simulink model "eq_test"  (Simulink 5.1)
settings: Solver=FixedStepDiscrete  StartTime=0.0  StopTime=inf  RelTol=1e-3
PreLoadFcn:
  | Frame=64;  % number of points in a frame
  | load eq_coefficients;
values from neighbouring files (symbols this model uses):
  D = 2 * W2 * (G01 - sqrt(G00 * G11))    [peq.m]
  num_den_coef = [0.998343259442 -1.98599942437 0.988847189128 1 -1.98599942437 0.98719044857 0.939478810291 -1.81918066061 0.879941563044 1 -1.81918066061 0.819420373336 ... (31 elements, 1x31)]    [eq_coefficients.mat]
undefined symbols (not defined in the file or in its folder): magnitude
libraries: dspsigops x4, dspsigattribs x3, dspsrcs4 x2, dspwin32 x2, dspbuff3 x2, dsparch3 x2, dspxfrm3 x2, dsparch4 x1, simulink x1
settings Model: Creator=aanantha  LastModifiedBy=dbenson  DataSet=allH.mat  SaveTime=off  SaveOutput=off  BooleanDataType=on  ProdHWDeviceType=Microprocessor  RTWOptions="-aEnforceIntegerDowncast=1 -aExtMode=0 -aExtModeTesting=0 -aFoldNonRolledExpr=1 -aForceParamTrailComments=0 -aGenerateComments=1 -aGenerateReport=0 -aIgnoreCustomStorageClasses=1 -aIncDataTypeInIds=0 -aIncHierarchyInIds=0 -aInlineInvariantSignals=0 -aInlinedPrmAccess=\"Literals\" -aLocalBlockOutputs=1 -aLogVarNameModifier=\"rt_\" -aMaxRTWIdLen=31 -aPrefixModelToSubsysFcnNames=1 -aRTWVerbose=1 -aRollThreshold=5 -aShowEliminatedStatements=0"

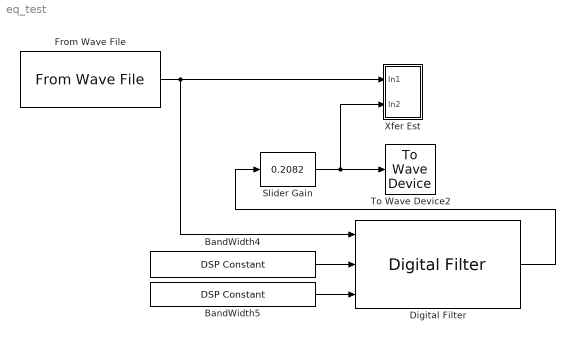
== system eq_test ==
  BandWidth4 : dspsrcs4/DSP Constant  Tag=paramsBlock  Value=conv(conv(num_den_coef(1:3),num_den_coef(7:9)),num_den_coef(13:15))  SampleMode=Discrete  discreteOutput=Sample-based  continuousOutput=Sample-based  sampTime=-1  framePeriod=-1  dataType=Inherit from 'Constant value'  wordLen=16  udDataType=sfix(16)  fracBitsMode=Best precision  numFracBits=15  InterpretAs1D=off  Ts=-1  FramebasedOutput=off
      settings: AttributesFormatString=\n\n\n\n
  BandWidth5 : dspsrcs4/DSP Constant  Tag=paramsBlock  Value=conv(conv(num_den_coef(4:6),num_den_coef(10:12)),num_den_coef(16:18))  SampleMode=Discrete  discreteOutput=Sample-based  continuousOutput=Sample-based  sampTime=-1  framePeriod=-1  dataType=Inherit from 'Constant value'  wordLen=16  udDataType=sfix(16)  fracBitsMode=Best precision  numFracBits=15  InterpretAs1D=off  Ts=-1  FramebasedOutput=off
      settings: AttributesFormatString=\n\n\n\n
  Digital Filter : dsparch4/Digital Filter  TypePopup=IIR (poles & zeros)  IIRFiltStruct=Direct form II transposed  AllPoleFiltStruct=Direct form  FIRFiltStruct=Direct form  CoeffSource=Input port(s)  NumCoeffs=[1 2]  DenCoeffs=[1 0.1]  BiQuadCoeffs=[1 0.3 0.4 1 0.1 0.2]  LatticeCoeffs=[0.2 0.4]  denIgnore=on  FiltPerSampPopup=One filter per frame  IC=0  ICnum=0  ICden=0  roundingMode=Floor  overflowMode=off
  From Wave File : dspwin32/From Wave File  FileName=test_wave.wav  SamplesPerFrame=Frame  MinBufSize=256  dType=Double  bLoop=on  timesToPlay=inf  restartMode=at beginning of next frame (zero pad)  firstSampleOutput=off  lastSampleOutput=off
  Slider Gain : simulink/Math Operations/Slider Gain  low=0.1  gain=0.2082  high=1
  To Wave Device2 : dspwin32/To Wave Device  bufDuration=2  initDelay=0.1  useDefaultDevice=off  userDeviceID=SoundMAX Digital Audio  enable24Bit=off
  Xfer Est : Subsystem  TreatAsAtomicUnit=on  mask(Xfer Scope){ScopeProperties=on, Domain=Frequency, HorizSpan=1, UseBuffer=on, BufferSize=512, Overlap=256, inpFftLenInherit=off, FFTlength=512, numAvg=4, DisplayProperties=off, AxisGrid=on, Memory=off, FrameNumber=on, AxisLegend=off, AxisZoom=off, OpenScopeAtSimStart=on, OpenScopeImmediately=off, FigPos=[484 458 442 191], AxisProperties=off, XUnits=Hertz, XRange=[0...Fs/2], InheritXIncr=on, XIncr=1, XLabel=Samples, YUnits=dB, YMin=-20, YMax=20, YLabel=Magnitude, dB, LineProperties=off, LineDisables=, LineStyles=, LineMarkers=, LineColors=[1 0 0]}
      mask prompts: ScopeProperties "_______ Scope properties _______"; Domain "Input domain:"; HorizSpan "Time display span (number of frames):"; UseBuffer "Buffer input"; BufferSize "Buffer size:"; Overlap "Buffer overlap:"; inpFftLenInherit "Specify FFT length"; FFTlength "FFT length:"; numAvg "Number of spectral averages:"; DisplayProperties "_______ Display properties _______"; AxisGrid "Show grid"; Memory "Persistence"; FrameNumber "Frame number"; AxisLegend "Channel legend"; AxisZoom "Compact display"; OpenScopeAtSimStart "Open scope at start of simulation"; OpenScopeImmediately "Open scope immediately"; FigPos "Scope position:"; AxisProperties "_______ Axis properties _______"; XUnits "Frequency units:"; XRange "Frequency range:"; InheritXIncr "Inherit sample increment from input"; XIncr "Sample time of original time series:"; XLabel "X-axis title:"; YUnits "Amplitude scaling:"; YMin "Minimum Y-limit:"; YMax "Maximum Y-limit:"; YLabel "Y-axis title:"; LineProperties "_______ Line properties _______"; LineDisables "Line visibility:"; LineStyles "Line styles:"; LineMarkers "Line markers:"; LineColors "Line colors:"
      mask help:
      | Computes a non-biased transfer function estimation by using
      | the ratio of the cross spectrum between the excitation and response
      | channels, and the autospectrum of the excitation channel.
      |
      | X= channel 1 = DUT excitation (discrete time random noise is best)
      | Y= channel 2 = DUT response from DUT
      |
      | Displays xfer function magnitude in linear or dB format.
      mask init:
      | [x,y,str] = xferscope1('icon');
      | s = xferscope1('init');
      settings: CopyFcn=sdspfscope2([],[],[],'BlockCopy');  DeleteFcn=sdspfscope2([],[],[],'BlockDelete');  NameChangeFcn=sdspfscope2([],[],[],'NameChange');  RTWSystemCode=Function
      mask Help:
      | Use a broad band discrete time excitation and apply it to both
      | analyzer the upper input port and the (discrete time) Device Under Test input.
      | Connect the discrete time DUT response to the lower input port.
      | Averaging of circa 100 produces good results.
      | 
      | The measurement results will be unbiased as long as the excitation
      | does not have noise which is correlated with noise in the response channel.
      | 
      | 
      | RAB 01/28/02
      mask StyleString: checkbox,popup(Time|Frequency|User-defined),edit,checkbox,edit,edit,checkbox,edit,edit,checkbox,checkbox,checkbox,checkbox,checkbox,checkbox,checkbox,checkbox,edit,checkbox,popup(Hertz|rad/sec),popup([0...Fs/2]|[-Fs/2...Fs/2]|[0...Fs]),checkbox,edit,edit,popup(Magnitude|dB),edit,edit,edit,checkbox,edit,edit,edit,edit
      mask CallbackString: dspblkbfftscope2('dynamic','ScopeProperties')|||dspblkbfftscope2('dynamic','useBuffer');|||dspblkbfftscope2('dynamic','FftLenCheckbox');|||dspblkbfftscope2('dynamic','DisplayProperties');|||||||dspblkbfftscope2('dynamic','OpenScope');||dspblkbfftscope2('dynamic','AxisProperties');|||dspblkbfftscope2('dynamic','InheritXIncr');|||||||dspblkbfftscope2('dynamic','LineProperties');||||
      mask Display: plot(x,y); text(14,20,str);
  wires:
  From Wave File/1 -> Digital Filter/1, Xfer Est/1(In1)
  Slider Gain/1 -> Xfer Est/2(In2), To Wave Device2/1
  BandWidth4/1 -> Digital Filter/2
  BandWidth5/1 -> Digital Filter/3
  Digital Filter/1 -> Slider Gain/1

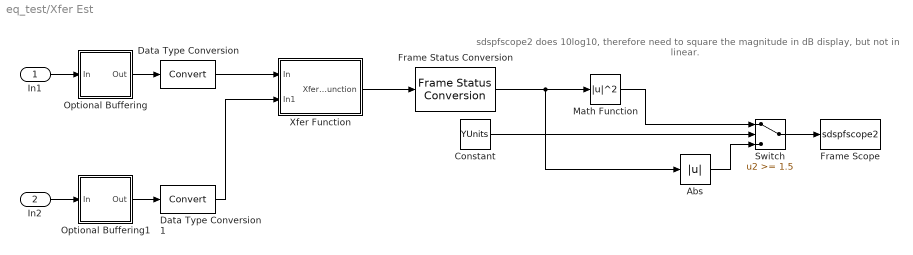
== system eq_test/Xfer Est ==
  note: sdspfscope2 does 10log10, therefore need to square the magnitude in dB
      | display, but not in linear.
  In1 : Inport
  In2 : Inport  Port=2
  Abs : Abs  SaturateOnIntegerOverflow=on
  Constant : Constant  Value=YUnits
  Data Type Conversion : DataTypeConversion  DataType=double  SaturateOnIntegerOverflow=on
  Data Type Conversion1 : DataTypeConversion  DataType=double  SaturateOnIntegerOverflow=on
  Frame Scope : S-Function  FunctionName=sdspfscope2  Parameters=s
  Frame Status Conversion : dspsigattribs/Frame Status Conversion  growRefPort=off  outframe=Sample-based
  Math Function : Math  Operator=magnitude^2
  Optional Buffering : Subsystem  mask(Replaceable Contents){oname=Buffer, osrc=dspbuff3/Buffer, oargs={'N','BufferSize','V','Overlap','ic','0'}, replace=strcmp(UseBuffer,'off')}
      mask prompts: oname "Relative name of blocks to replace:"; osrc "Simulink path to each source block:"; oargs "Parameter/value pairs to each block:"; replace "Replace with short-circuit:"
      mask help: Configurable subsystem holding blocks which may be replaced by virtual short-circuits (muxes) when not needed.
      mask init:
      | opts.name = oname; opts.src = osrc; opts.args = oargs;
      | dspskipblk(gcb,opts,replace);
  Optional Buffering1 : Subsystem  mask(Replaceable Contents){oname=Buffer, osrc=dspbuff3/Buffer, oargs={'N','BufferSize','V','Overlap','ic','0'}, replace=strcmp(UseBuffer,'off')}
      mask prompts: oname "Relative name of blocks to replace:"; osrc "Simulink path to each source block:"; oargs "Parameter/value pairs to each block:"; replace "Replace with short-circuit:"
      mask help: Configurable subsystem holding blocks which may be replaced by virtual short-circuits (muxes) when not needed.
      mask init:
      | opts.name = oname; opts.src = osrc; opts.args = oargs;
      | dspskipblk(gcb,opts,replace);
  Switch : Switch  Threshold=1.5  SaturateOnIntegerOverflow=on  InputSameDT=on
  Xfer Function : Subsystem  mask(Xfer Function){wintype=Hann, Rs=50, beta=5, winsamp=Periodic, inheritFFT=on, fftsize=FFTlength, navg=numAvg}
      mask prompts: wintype "Window type:"; Rs "Stopband attenuation in dB:"; winsamp "Window sampling:"; inheritFFT "Inherit FFT length from input dimensions"; fftsize "FFT length:"; navg "Number of spectral averages:"
      mask init:
      | [x,y,xe]=Xfer_Function1('icon');
      | Xfer_Function1('init');
      mask StyleString: popup(Bartlett|Blackman|Boxcar|Chebyshev|Hamming|Hann|Hanning|Kaiser|Triang),edit,edit,popup(Symmetric|Periodic),checkbox,edit,edit
      mask CallbackString: dspblkshorttimefft2||||dspblkshorttimefft2||
      mask Display: text(-3,1.15,'Xfer_Function'); plot((-xe),0,xe,1.3,x,y)
  wires:
  Constant/1 -> Switch/2
  Switch/1 -> Frame Scope/1
  Math Function/1 -> Switch/1
  Data Type Conversion1/1 -> Xfer Function/2(In1)
  Optional Buffering1/1(Out) -> Data Type Conversion1/1
  In2/1 -> Optional Buffering1/1(In)
  Frame Status Conversion/1 -> Abs/1, Math Function/1
  Xfer Function/1(Xfer_Function) -> Frame Status Conversion/1
  In1/1 -> Optional Buffering/1(In)
  Optional Buffering/1(Out) -> Data Type Conversion/1
  Data Type Conversion/1 -> Xfer Function/1(In)
  Abs/1 -> Switch/3

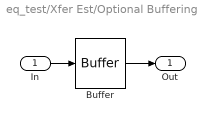
== system eq_test/Xfer Est/Optional Buffering ==
  In : Inport
  Buffer : dspbuff3/Buffer  N=BufferSize  V=Overlap  ic=0
  Out : Outport  InitialOutput=0
  wires:
  Buffer/1 -> Out/1
  In/1 -> Buffer/1

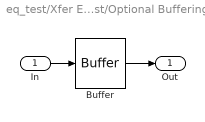
== system eq_test/Xfer Est/Optional Buffering1 ==
  In : Inport
  Buffer : dspbuff3/Buffer  N=BufferSize  V=Overlap  ic=0
  Out : Outport  InitialOutput=0
  wires:
  In/1 -> Buffer/1
  Buffer/1 -> Out/1

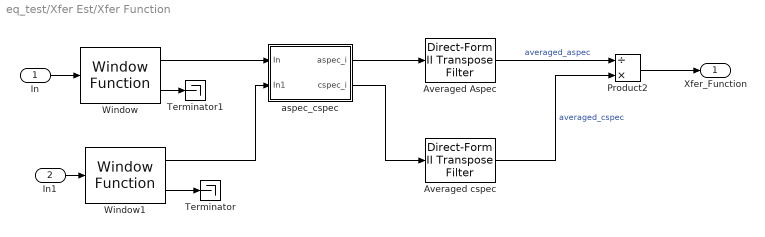
== system eq_test/Xfer Est/Xfer Function ==
  In : Inport
  In1 : Inport  Port=2
  "Averaged Aspec " : dsparch3/Direct-Form II Transpose Filter  num=1  den=[abs(navg) ,-(abs(navg)-1)]  ic=eps
  Averaged cspec : dsparch3/Direct-Form II Transpose Filter  num=1  den=[abs(navg),-(abs(navg)-1)]  ic=eps
  Product2 : Product  Inputs=/*  SaturateOnIntegerOverflow=on  InputSameDT=on
  Terminator : Terminator
  Terminator1 : Terminator
  Window : dspsigops/Window Function  winmode=Generate and apply window  wintype=Hann  sampmode=Continuous  samptime=1  N=64  Rs=Rs  beta=beta  winsamp=Periodic  UserWindow=hamming  OptParams=off  UserParams={1.0}  dataType=double  wordLen=16  udDataType=sfix(16)  fracBitsMode=Best precision  numFracBits=15  roundingMode=Floor  overflowMode=off
  Window1 : dspsigops/Window Function  winmode=Generate and apply window  wintype=Hann  sampmode=Continuous  samptime=1  N=64  Rs=Rs  beta=beta  winsamp=Symmetric  UserWindow=hamming  OptParams=off  UserParams={1.0}  dataType=double  wordLen=16  udDataType=sfix(16)  fracBitsMode=Best precision  numFracBits=15  roundingMode=Floor  overflowMode=off
  aspec_cspec : Subsystem  mask(aspec_aspec){fftLenInherit=on, fftsize=fftsize}
      mask prompts: fftLenInherit "Inherit FFT length from input dimensions"; fftsize "FFT length:"
      mask init:
      | aspec_cspec1('init');aspec_cspec1('update'); str='aspec_cspec';
      mask CallbackString: dspblkmagfft2;|
      mask Display: disp(str);
  Xfer_Function : Outport  InitialOutput=0
  wires:
  Averaged cspec/1 -> Product2/2  "averaged_cspec"
  Window/2 -> Terminator1/1
  aspec_cspec/2(cspec_i) -> Averaged cspec/1
  Window1/2 -> Terminator/1
  Window1/1 -> aspec_cspec/2(In1)
  In1/1 -> Window1/1
  In/1 -> Window/1
  aspec_cspec/1(aspec_i) -> "Averaged Aspec "/1
  Window/1 -> aspec_cspec/1(In)
  Product2/1 -> Xfer_Function/1
  "Averaged Aspec "/1 -> Product2/1  "averaged_aspec"

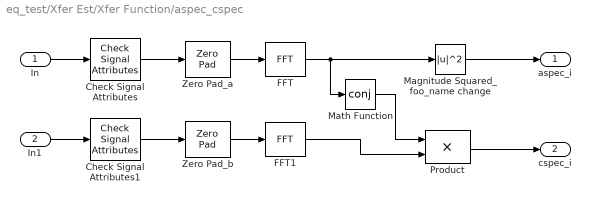
== system eq_test/Xfer Est/Xfer Function/aspec_cspec ==
  In : Inport
  In1 : Inport  Port=2
  Check Signal Attributes : dspsigattribs/Check Signal Attributes  SigAttribCheckMethod=Matches attributes exactly  Complexity=Ignore  Frame=Sample-based  DimsCheckMethod=Is...  Dimensions=Row vector (2-D)  DatatypeCheckMethod=Ignore  DatatypeGeneral=Boolean  DtypeFloatSpecific=Any floating-point  DtypeFixedSpecific=Any fixed-point  DtypeIntSpecific=Any integer  SampleMode=Ignore
  Check Signal Attributes1 : dspsigattribs/Check Signal Attributes  SigAttribCheckMethod=Matches attributes exactly  Complexity=Ignore  Frame=Sample-based  DimsCheckMethod=Is...  Dimensions=Row vector (2-D)  DatatypeCheckMethod=Ignore  DatatypeGeneral=Boolean  DtypeFloatSpecific=Any floating-point  DtypeFixedSpecific=Any fixed-point  DtypeIntSpecific=Any integer  SampleMode=Ignore
  FFT : dspxfrm3/FFT  CompMethod=Table lookup  TableOpt=Speed  BitRevOrder=off  SkipNorm=off  firstCoeffMode=User-defined  firstCoeffWordLength=16  firstCoeffFracLength=15  roundingMode=Floor  overflowMode=off
  FFT1 : dspxfrm3/FFT  CompMethod=Table lookup  TableOpt=Speed  BitRevOrder=off  SkipNorm=off  firstCoeffMode=User-defined  firstCoeffWordLength=16  firstCoeffFracLength=15  roundingMode=Floor  overflowMode=off
  Magnitude Squared_foo_name change : Math  Operator=magnitude^2
  Math Function : Math  Operator=conj
  Product : Product  SaturateOnIntegerOverflow=on  InputSameDT=on
  Zero Pad_a : dspsigops/Zero Pad  padSigAt=End  zpadAlong=None  padNumOutRowsSpecMethod=User-specified  numOutRows=fftsize  padNumOutColsSpecMethod=User-specified  numOutCols=1  trunc_flag=None
  Zero Pad_b : dspsigops/Zero Pad  padSigAt=End  zpadAlong=None  padNumOutRowsSpecMethod=User-specified  numOutRows=fftsize  padNumOutColsSpecMethod=User-specified  numOutCols=1  trunc_flag=None
  aspec_i : Outport
  cspec_i : Outport  Port=2
  wires:
  Product/1 -> cspec_i/1
  FFT1/1 -> Product/2
  Math Function/1 -> Product/1
  Zero Pad_b/1 -> FFT1/1
  Check Signal Attributes1/1 -> Zero Pad_b/1
  In1/1 -> Check Signal Attributes1/1
  Magnitude Squared_foo_name change/1 -> aspec_i/1
  In/1 -> Check Signal Attributes/1
  FFT/1 -> Magnitude Squared_foo_name change/1, Math Function/1
  Zero Pad_a/1 -> FFT/1
  Check Signal Attributes/1 -> Zero Pad_a/1
